simulink model "PP_NLE"  (R2024b)
settings: Solver=VariableStepAuto  StartTime=0.0  StopTime=10.0  RelTol=1e-3
values from neighbouring files (symbols this model uses):
  disorder_times = [15, 16]    [exam.m]    (also in exam2.m; exam3.m = [12, 16]; exam4.m = [15, 25]; practical_exam_assignment3.m = [30, 40])
undefined symbols (not defined in the file or in its folder): K, N
settings Model: Creator=lukiq  LastModifiedBy=lukiq
settings DebuggingCC: AlgebraicLoopMsg=none

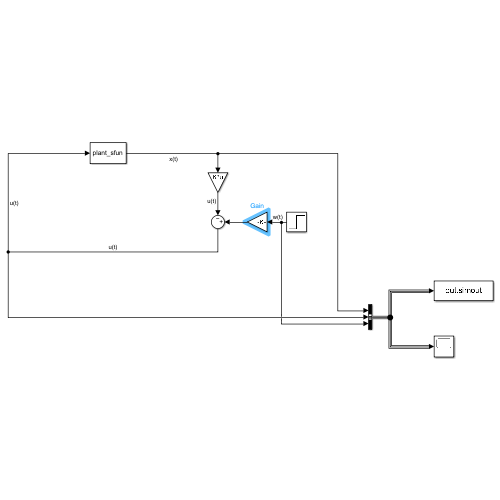
[thumbnail: Simulink's stored preview of the top-level diagram]
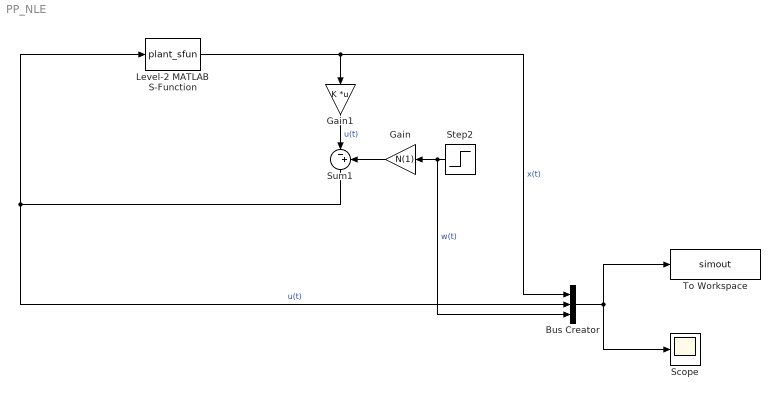
== system PP_NLE ==
  Bus Creator : BusCreator  Inputs=3
  Gain : Gain  Gain=N(1)
  Gain1 : Gain  Gain=K  Multiplication=Matrix(K*u)
  Level-2 MATLAB S-Function : M-S-Function  FunctionName=plant_sfun  Parameters=odeHandleSimulink, p, u, outIdx
  Scope : Scope
  Step2 : Step  Time=disorder_times(1)  SampleTime=0
  Sum1 : Sum  Inputs=|-+
  To Workspace : ToWorkspace  VariableName=simout  SaveFormat=Timeseries  SampleTime=-1
  wires:
  Sum1/1 -> Level-2 MATLAB S-Function/1, Bus Creator/2  "u(t)"
  Bus Creator/1 -> Scope/1, To Workspace/1
  Gain1/1 -> Sum1/1  "u(t)"
  Step2/1 -> Bus Creator/3, Gain/1  "w(t)"
  Level-2 MATLAB S-Function/1 -> Gain1/1, Bus Creator/1  "x(t)"
  Gain/1 -> Sum1/2
